simulink model "Task_30"  (R2022b)
settings: Solver=VariableStepAuto  StartTime=0.0  StopTime=10.0  RelTol=1e-3
settings Model: Creator=Abanob_Sameh  LastModifiedBy=Abanob_Sameh

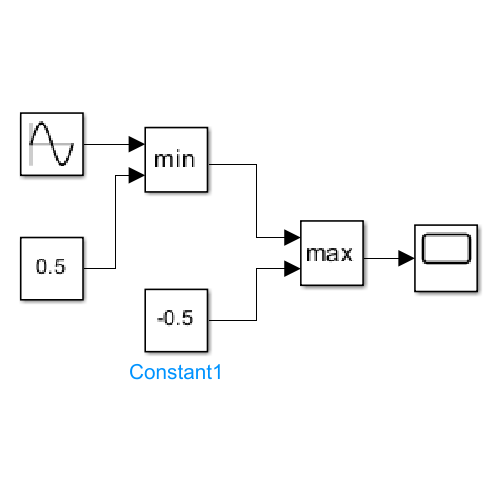
[thumbnail: Simulink's stored preview of the top-level diagram]
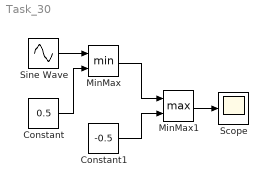
== system Task_30 ==
  Constant : Constant  Value=0.5
  Constant1 : Constant  Value=-0.5
  MinMax : MinMax  Inputs=2
  MinMax1 : MinMax  Function=max  Inputs=2
  Scope : Scope
  Sine Wave : Sin  SampleTime=0
  wires:
  Sine Wave/1 -> MinMax/1
  MinMax/1 -> MinMax1/1
  Constant/1 -> MinMax/2
  Constant1/1 -> MinMax1/2
  MinMax1/1 -> Scope/1
